simulink subsystem "ManipulatorMechanicsSubsystem"  (R2023a)
settings: Solver=VariableStepAuto  StartTime=0.0  StopTime=10.0  RelTol=1e-3
undefined symbols (not defined in the file or in its folder): app, DiscIntNeverNeededParam, Generate_B, GenerateGeometricJacobian, TrimUnusedDofs_rows
settings Model: Creator=Ericw  LastModifiedBy=Ericw

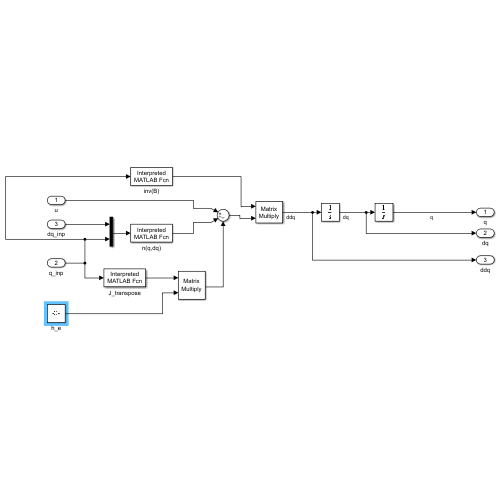
[thumbnail: Simulink's stored preview of the top-level diagram]
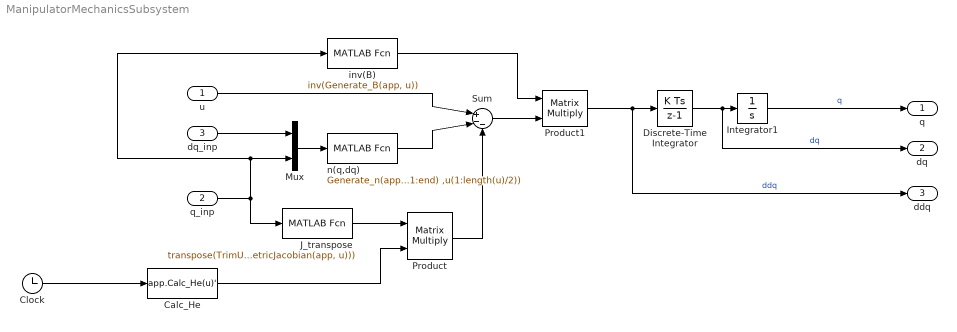
== system ManipulatorMechanicsSubsystem ==
  u : Inport  PortDimensions=[app.NumJoints,1]
  q_inp : Inport  Port=2  PortDimensions=[app.NumJoints,1]
  dq_inp : Inport  Port=3  PortDimensions=[app.NumJoints,1]
  Calc_He : MATLABFcn  MATLABFcn=app.Calc_He(u)'  OutputDimensions=[app.numActiveDofs,1]  Output1D=off
  Clock : Clock
  Discrete-Time Integrator : DiscreteIntegrator  InitialCondition=zeros(app.NumJoints,1)  SampleTime=-1  ICPrevOutput=DiscIntNeverNeededParam  ICPrevScaledInput=DiscIntNeverNeededParam
  Integrator1 : Integrator  InitialCondition=app.q_0_i
  J_transpose : MATLABFcn  MATLABFcn=transpose(TrimUnusedDofs_rows(app,GenerateGeometricJacobian(app, u)))  OutputDimensions=[app.NumJoints,app.numActiveDofs]  Output1D=off
  Mux : Mux  Inputs=2
  Product : Product  Multiplication=Matrix(*)
  Product1 : Product  Multiplication=Matrix(*)
  Sum : Sum  Inputs=|+--
  inv(B) : MATLABFcn  MATLABFcn=inv(Generate_B(app, u))  OutputDimensions=[app.NumJoints,app.NumJoints]  Output1D=off
  n(q,dq) : MATLABFcn  MATLABFcn=Generate_n(app,u(length(u)/2+1:end) ,u(1:length(u)/2))  OutputDimensions=[app.NumJoints,1]  Output1D=off
  q : Outport  PortDimensions=[app.NumJoints,1]
  dq : Outport  Port=2  PortDimensions=[app.NumJoints,1]
  ddq : Outport  Port=3  PortDimensions=[app.NumJoints,1]
  wires:
  u/1 -> Sum/1
  q_inp/1 -> Mux/2, inv(B)/1, J_transpose/1
  J_transpose/1 -> Product/1
  Calc_He/1 -> Product/2
  Product/1 -> Sum/3
  dq_inp/1 -> Mux/1
  Mux/1 -> n(q,dq)/1
  n(q,dq)/1 -> Sum/2
  inv(B)/1 -> Product1/1
  Sum/1 -> Product1/2
  Integrator1/1 -> q/1  "q"
  Discrete-Time Integrator/1 -> Integrator1/1, dq/1  "dq"
  Product1/1 -> Discrete-Time Integrator/1, ddq/1  "ddq"
  Clock/1 -> Calc_He/1
